simulink model "f22pil"  (Simulink 3.00)
settings: Solver=ode45  StartTime=data.time(1)  StopTime=data.time(end)  RelTol=1e-3
libraries: smxl x7, pil x2
settings Model: BooleanDataType=on  RTWOptions="-aEnforceIntegerDowncast=1 -aFoldNonRolledExpr=1 -aInlineInvariantSignals=0 -aInlineParameters=0 -aLocalBlockOutputs=1 -aRollThreshold=5 -aZeroInternalMemoryAtStartup=1 -aZeroExternalMemoryAtStartup=1 -aInitFltsAndDblsToZero=1 -aGenerateReport=0 -aGenCodeOnly=0 -aRTWVerbose=1 -aIncludeHyperlinkInReport=0 -aLaunchReport=0 -aForceParamTrailComments=0 -aGenerateComments=1 -aIgnoreCustomStorageClasses=1 -aIncHierarchyInIds=0 -aMaxRTWIdLen=31 -aShowEliminatedStatements=0 -aPrefixModelToSubsysFcnNames=1 -aIncDataTypeInIds=0 -aInsertBlockDesc=0 -aSimulinkBlockComments=1 -aInlinedPrmAccess=\"Literals\"  -aSuppressErrorStatus=0 -aModelReferenceCompliant=1 -aSupportNonInlinedSFcns=1 -aSupportContinuousTime=1 -aSupportComplex=1 -aSupportNonFinite=1 -aSupportAbsoluteTime=1 -aTargetFcnLib=\"ansi_tfl_tmw.mat\" -aMultiInstanceERTCode=0 -aLogVarNameModifier=\"rt_\" -aIsPILTarget=0 -aCombineOutputUpdateFcns=0 -aGenerateASAP2=0 -aGenerateSampleERTMain=0 -aGenerateFullHeader=1 -aUtilityFuncGeneration=\"Auto\" -aIncludeFileDelimiter=\"Auto\" -aIncludeMdlTerminateFcn=1 -aPurelyIntegerCode=0 -aERTCustomFileBanners=0 -aRTWCAPIStates=0 -aRTWCAPIParams=0 -aRTWCAPISignals=0 -aMatFileLogging=1 -aGenFloatMathFcnCalls=\"ANSI_C\" -aExtModeMexFile=\"ext_comm\" -aExtModeTransport=0 -aExtModeStaticAllocSize=1000000 -aExtModeTesting=0 -aExtModeStaticAlloc=0 -aExtMode=0"  ExtModeTrigMode=normal  ExtModeArmWhenConnect=on  Creator=Karebear  LastModifiedBy=sim

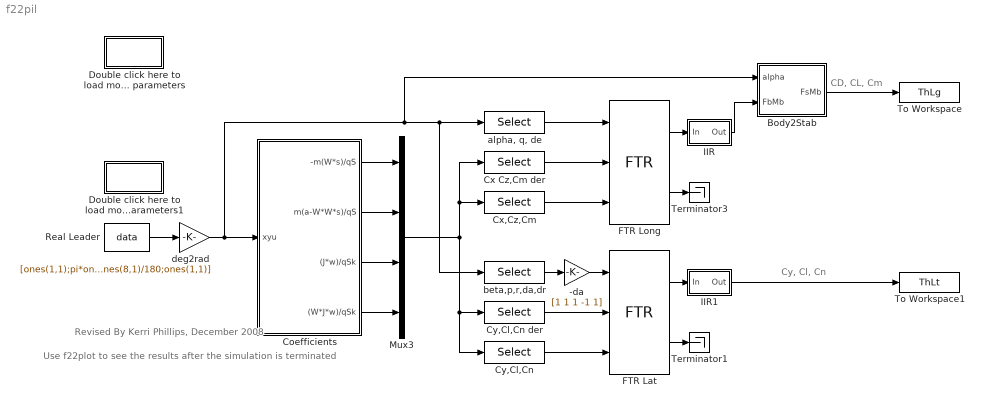
== system f22pil ==
  note: CD, CL, Cm
  note: Cy, Cl, Cn
  note: Revised By Kerri Phillips,
      | December 2008
  note: Use f22plot to see the results
      | after the simulation is terminated
  -da : Gain  Gain=[1 1 1 -1 1]  SaturateOnIntegerOverflow=on
  Body2Stab : Subsystem
  Coefficients : Subsystem
  Cx Cz,Cm der : Selector  Elements=[1 3 8]  InputPortWidth=12
  Cx,Cz,Cm : Selector  Elements=[4 6 11]  InputPortWidth=12
  Cy,Cl,Cn : Selector  Elements=[5 10 12]  InputPortWidth=12
  Cy,Cl,Cn der : Selector  Elements=[2 7 9]  InputPortWidth=12
  Double click here to load model and parameters : Subsystem
      settings: OpenFcn=load f22data;
      mask Display: disp('Load\nData')
  Double click here to load model and parameters1 : Subsystem
      mask Display: disp('Signals')
  FTR Lat : pil/Theta & Cov/FTR  ths=[5 3]  w=2*pi*linspace(0.2,2,30)'  T=0.02
  FTR Long : pil/Theta & Cov/FTR  ths=[3 3]  w=2*pi*linspace(0.2,2,30)'  T=0.02
  IIR : Subsystem  mask(Discrete Time First Order IIR){ni=3*3, a=1, x0=0, T=0.02}
      mask prompts: ni "Number of Channels"; a "Cutoff Frequency (a)"; x0 "Initial Condition"; T "Sample Time"
      mask help:
      | Each channel has the transfer function
      |   (1-exp(-aT))/(1-exp(-aT)(z^-1)) which is a
      |   good approximation of a/(s+a) if 4*pi*a*T<1
      mask init:
      | A=[];B=[];C=[];D=[];
      | for i=1:ni,
      | A=[A,zeros(size(A,1),1);zeros(1,size(A,2)),exp(-a*T)];
      | B=[B,zeros(size(B,1),1);zeros(1,size(B,2)),1-exp(-a*T)];
      | C=[C,zeros(size(C,1),1);zeros(1,size(C,2)),exp(-a*T)];
      | D=[D,zeros(size(D,1),1);zeros(1,size(D,2)),1-exp(-a*T)];
      | end
      mask Help:
      | <p>
      |   Each channel has the transfer function
      |   (1-exp(-aT))/(1-exp(-aT)(z^-1)) which is a
      |   good approximation of a/(s+a) if 4*pi*a*T<1
      | </p>
      mask Display: disp('a/(s+a)')
  IIR1 : Subsystem  mask(Discrete Time First Order IIR){ni=5*3, a=1, x0=0, T=0.02}
      mask prompts: ni "Number of Channels"; a "Cutoff Frequency (a)"; x0 "Initial Condition"; T "Sample Time"
      mask help:
      | Each channel has the transfer function
      |   (1-exp(-aT))/(1-exp(-aT)(z^-1)) which is a
      |   good approximation of a/(s+a) if 4*pi*a*T<1
      mask init: same as f22pil/IIR
      mask Help:
      | <p>
      |   Each channel has the transfer function
      |   (1-exp(-aT))/(1-exp(-aT)(z^-1)) which is a
      |   good approximation of a/(s+a) if 4*pi*a*T<1
      | </p>
      mask Display: disp('a/(s+a)')
  Mux3 : Mux  Inputs=[3 3 3 3]
  Real Leader : FromWorkspace  VariableName=data  SampleTime=0.02  HoldFinalValue=off
  Terminator1 : Terminator
  Terminator3 : Terminator
  To Workspace : ToWorkspace  VariableName=ThLg  SampleTime=0.02  SaveFormat=Matrix
      settings: Buffer=1000
  To Workspace1 : ToWorkspace  VariableName=ThLt  SampleTime=0.02  SaveFormat=Matrix
      settings: Buffer=1000
  "alpha, q, de" : Selector  Elements=[2 5 19]  InputPortWidth=27
  beta,p,r,da,dr : Selector  Elements=[3 4 6 21 23]  InputPortWidth=27
  deg2rad : Gain  Gain=[ones(1,1);pi*ones(8,1)/180;ones(9,1);pi*ones(8,1)/180;ones(1,1)]  SaturateOnIntegerOverflow=on
  wires:
  Real Leader/1 -> deg2rad/1
  deg2rad/1 -> Coefficients/1(xyu), "alpha, q, de"/1, beta,p,r,da,dr/1, Body2Stab/1(alpha)
  "alpha, q, de"/1 -> FTR Long/1
  Cx Cz,Cm der/1 -> FTR Long/2
  Cx,Cz,Cm/1 -> FTR Long/3
  Coefficients/1(-m(W*s)/qS) -> Mux3/1
  Coefficients/2(m(a-W*W*s)/qS) -> Mux3/2
  Coefficients/3((J*w)/qSk) -> Mux3/3
  Coefficients/4((W*J*w)/qSk) -> Mux3/4
  Cy,Cl,Cn der/1 -> FTR Lat/2
  Cy,Cl,Cn/1 -> FTR Lat/3
  Mux3/1 -> Cx Cz,Cm der/1, Cx,Cz,Cm/1, Cy,Cl,Cn/1, Cy,Cl,Cn der/1
  beta,p,r,da,dr/1 -> -da/1
  FTR Long/2 -> Terminator3/1
  FTR Lat/2 -> Terminator1/1
  FTR Long/1 -> IIR/1(In)
  FTR Lat/1 -> IIR1/1(In)
  IIR1/1(Out) -> To Workspace1/1
  -da/1 -> FTR Lat/1
  Body2Stab/1(FsMb) -> To Workspace/1
  IIR/1(Out) -> Body2Stab/2(FbMb)

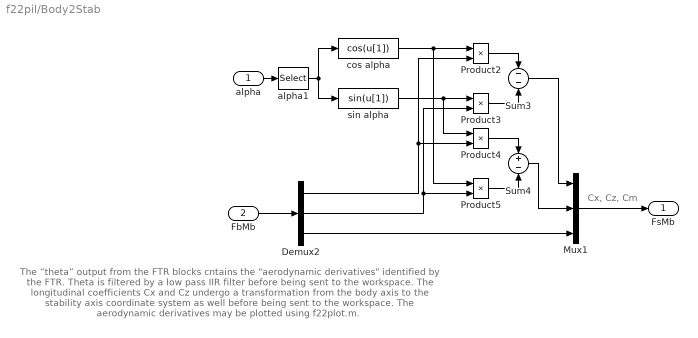
== system f22pil/Body2Stab ==
  note: Cx, Cz, Cm
  note: The “theta” output from the FTR blocks cntains the "aerodynamic derivatives" identified by the FTR.
      | Theta is filtered by a low pass IIR filter before being sent to the workspace.
      | The longitudinal coefficients Cx and Cz undergo a transformation from the body axis
      | to the stability axis coordinate system as well before being sent to the workspace.
      | The aerodynamic derivatives may be plotted using f22plot.m.
  alpha : Inport  Port=1  PortWidth=-1  SampleTime=-1  DataType=auto
      settings: SignalType=auto
  FbMb : Inport  Port=2  PortWidth=-1  SampleTime=-1  DataType=auto
      settings: SignalType=auto
  Demux2 : Demux  Outputs=[3 3 3]
  Mux1 : Mux  Inputs=[3 3 3]
      settings: DisplayOption=none
  Product{2..5} (4 alike) : Product  Inputs=2  SaturateOnIntegerOverflow=on
  Sum3 : Sum  Inputs=--  SaturateOnIntegerOverflow=on
  Sum4 : Sum  Inputs=+-  SaturateOnIntegerOverflow=on
  alpha1 : Selector  Elements=2  InputPortWidth=27
  cos alpha : Fcn  Expr=cos(u[1])
  sin alpha : Fcn  Expr=sin(u[1])
  FsMb : Outport  Port=1
  wires:
  Mux1/1 -> FsMb/1
  Product5/1 -> Sum4/2
  Product4/1 -> Sum4/1
  Demux2/2 -> Product5/2, Product3/2
  sin alpha/1 -> Product4/1, Product3/1
  Product3/1 -> Sum3/2
  Product2/1 -> Sum3/1
  Demux2/1 -> Product4/2, Product2/2
  cos alpha/1 -> Product5/1, Product2/1
  alpha/1 -> alpha1/1
  Sum4/1 -> Mux1/2
  Sum3/1 -> Mux1/1
  Demux2/3 -> Mux1/3
  FbMb/1 -> Demux2/1
  alpha1/1 -> cos alpha/1, sin alpha/1

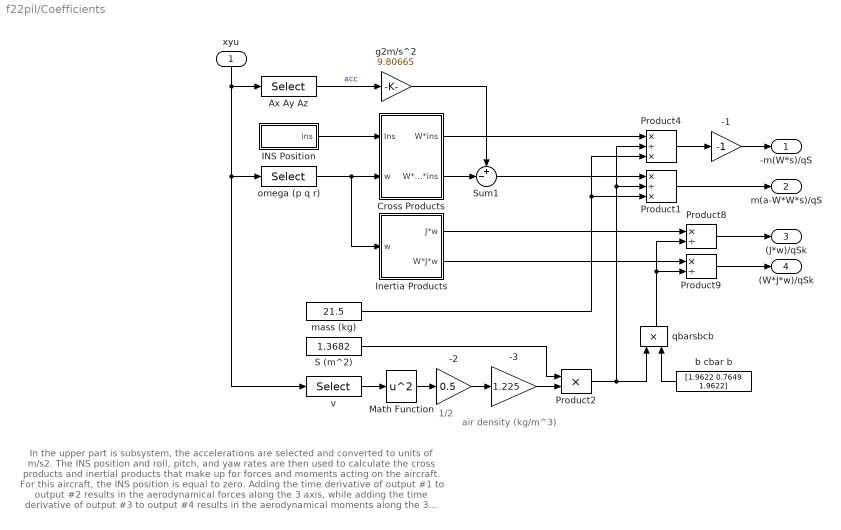
== system f22pil/Coefficients ==
  note: air density
      |  (kg/m^3)
  note: 1/2
  note: In the upper part is subsystem, the accelerations are selected and converted to units of m/s2.
      | The INS position and roll, pitch, and yaw rates are then used to calculate the cross products and inertial products that
      | make up for forces and moments acting on the aircraft. For this aircraft, the INS position is equal to zero.
      | Adding the time derivative of output #1 to output #2 results in the aerodynamical forces along the 3 axis,
      | while adding the time derivative of output #3 to output #4 results in the aerodynamical moments along the 3 axis.
  xyu : Inport  Orientation=down  Port=1  PortWidth=-1  SampleTime=-1  DataType=auto
      settings: SignalType=auto
  -1 : Gain  Gain=-1  SaturateOnIntegerOverflow=on
  -2 : Gain  Gain=0.5  SaturateOnIntegerOverflow=on
  -3 : Gain  Gain=1.225  SaturateOnIntegerOverflow=on
  Ax Ay Az : Selector  Elements=[16 17 18]  InputPortWidth=27
  Cross Products : Subsystem
  INS Position : Subsystem  mask(INS Position in Body Axes){inspos=[0 0 0], cgpos=[0 0 0]}
      mask prompts: inspos "INS Position in inches [FS,BL,WL]"; cgpos "CG  Position in inches [FS,BL,WL]"
      mask help:
      | This block gives in output the INS
      |   position in feets in body axes.
      |
      |   Both INS and CG positions are given
      |   in the mask as Fuselage Station, Butt Line,
      |   and Water Line measurements in inches.
      mask Help:
      | This block gives in output the INS
      |   position in feets in body axes.
      | 
      |   Both INS and CG positions are given
      |   in the mask as Fuselage Station, Butt Line,
      |   and Water Line measurements in inches.
  Inertia Products : Subsystem
  Math Function : Math  Operator=square  OutputSignalType=auto
  Product1 : Product  Inputs=*/*  SaturateOnIntegerOverflow=on
  Product2 : Product  Inputs=**  SaturateOnIntegerOverflow=on
  Product4 : Product  Inputs=*/*  SaturateOnIntegerOverflow=on
  Product8 : Product  Inputs=*/  SaturateOnIntegerOverflow=on
  Product9 : Product  Inputs=*/  SaturateOnIntegerOverflow=on
  S (m^2) : Constant  Value=1.3682
  Sum1 : Sum  Inputs=+-|  SaturateOnIntegerOverflow=on
  b cbar b : Constant  Orientation=left  Value="[1.9622    0.7649    1.9622]"
  g2m/s^2 : Gain  Gain=9.80665  SaturateOnIntegerOverflow=on
  mass (kg) : Constant  Value=21.5
  omega (p q r) : Selector  Elements=[4 5 6]  InputPortWidth=27
  qbarsbcb : Product  Orientation=up  Inputs=2  SaturateOnIntegerOverflow=on
  v : Selector  Elements=1  InputPortWidth=27
  -m(W*s)/qS : Outport  Port=1
  m(a-W*W*s)/qS : Outport  Port=2
  (J*w)/qSk : Outport  Port=3
  (W*J*w)/qSk : Outport  Port=4
  wires:
  Inertia Products/1(J*w) -> Product8/1
  Inertia Products/2(W*J*w) -> Product9/1
  Cross Products/2(W*W*ins) -> Sum1/2
  Product9/1 -> (W*J*w)/qSk/1
  Product8/1 -> (J*w)/qSk/1
  Product4/1 -> -1/1
  -1/1 -> -m(W*s)/qS/1
  Product1/1 -> m(a-W*W*s)/qS/1
  Sum1/1 -> Product1/1
  omega (p q r)/1 -> Inertia Products/1(w), Cross Products/2(w)
  Ax Ay Az/1 -> g2m/s^2/1  "acc"
  INS Position/1(ins) -> Cross Products/1(Ins)
  xyu/1 -> Ax Ay Az/1, omega (p q r)/1, v/1
  Cross Products/1(W*ins) -> Product4/1
  g2m/s^2/1 -> Sum1/1
  mass (kg)/1 -> Product4/3, Product1/3
  S (m^2)/1 -> Product2/1
  v/1 -> Math Function/1
  -2/1 -> -3/1
  Math Function/1 -> -2/1
  -3/1 -> Product2/2
  Product2/1 -> Product4/2, Product1/2, qbarsbcb/1
  qbarsbcb/1 -> Product8/2, Product9/2
  b cbar b/1 -> qbarsbcb/2

== system f22pil/Double click here to load model and parameters ==

== system f22pil/Double click here to load model and parameters1 ==
  note: 1.  Airspeed (m/s)
      | 2.  Angle of Attack (deg)
      | 3.  Sideslip Angle (deg)
      | 4.  Roll Rate (deg/s)
      | 5.  Pitch Rate (deg/s)
      | 6.  Yaw Rate (deg/s)
      | 7.  Yaw Angle (deg)
      | 8.  Pitch Angle (deg)
      | 9.  Roll Angle (deg)
      | 10 x GPS position (m)
      | 11. y GPS position (m)
      | 12. z GPS position (m)
      | 13. x GPS velocity (m/s)
      | 14. y GPS velocity (m/s)
      | 15. z GPS velocity (m/s)
      | 16. x Acceleration (g)
      | 17. y Acceleration (g)
      | 18. z Acceleration (g)
      | 19. Left Stabilator Deflection (deg)
      | 20. Right Stabilator Deflection (deg)
      | 21. Left Aileron Deflection (deg)
      | 22. Right Aileron Deflection (deg)
      | 23. Left Rudder Deflection (deg)
      | 24. Right Rudder Deflection (deg)
      | 25. Left Flap Deflection (deg)
      | 26. Right Flap Deflection (deg)
      | 27.Throttle Command

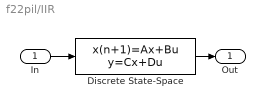
== system f22pil/IIR ==
  In : Inport  Port=1  PortWidth=-1  SampleTime=-1  DataType=auto
      settings: SignalType=auto
  Discrete State-Space : DiscreteStateSpace  A=A  B=B  C=C  D=D  X0=x0  SampleTime=T
  Out : Outport  Port=1
  wires:
  Discrete State-Space/1 -> Out/1
  In/1 -> Discrete State-Space/1

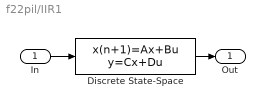
== system f22pil/IIR1 ==
  In : Inport  Port=1  PortWidth=-1  SampleTime=-1  DataType=auto
      settings: SignalType=auto
  Discrete State-Space : DiscreteStateSpace  A=A  B=B  C=C  D=D  X0=x0  SampleTime=T
  Out : Outport  Port=1
  wires:
  In/1 -> Discrete State-Space/1
  Discrete State-Space/1 -> Out/1

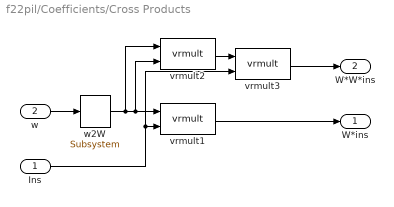
== system f22pil/Coefficients/Cross Products ==
  Ins : Inport  Port=1  PortWidth=-1  SampleTime=-1  DataType=auto
      settings: SignalType=auto
  w : Inport  Port=2  PortWidth=-1  SampleTime=-1  DataType=auto
      settings: SignalType=auto
  vrmult1 : smxl/Real Matrices/vrmult  dims=[3 3 1]
  vrmult2 : smxl/Real Matrices/vrmult  dims=[3 3 3]
  vrmult3 : smxl/Real Matrices/vrmult  dims=[3 3 1]
  w2W : smxl/Rotation Matrices/Quaternions/Body2Earth/Subsystem
  W*ins : Outport  Port=1
  W*W*ins : Outport  Port=2
  wires:
  Ins/1 -> vrmult3/2, vrmult1/2
  vrmult3/1 -> W*W*ins/1
  vrmult2/1 -> vrmult3/1
  vrmult1/1 -> W*ins/1
  w2W/1 -> vrmult2/2, vrmult1/1, vrmult2/1
  w/1 -> w2W/1

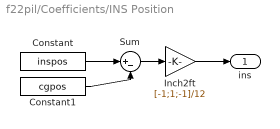
== system f22pil/Coefficients/INS Position ==
  Constant : Constant  Value=inspos
  Constant1 : Constant  Value=cgpos
  Inch2ft : Gain  Gain=[-1;1;-1]/12  SaturateOnIntegerOverflow=on
  Sum : Sum  Inputs=|+-  SaturateOnIntegerOverflow=on
  ins : Outport  Port=1
  wires:
  Inch2ft/1 -> ins/1
  Sum/1 -> Inch2ft/1
  Constant1/1 -> Sum/2
  Constant/1 -> Sum/1

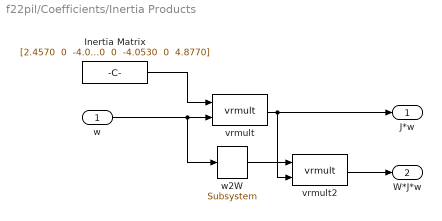
== system f22pil/Coefficients/Inertia Products ==
  w : Inport  Port=1  PortWidth=-1  SampleTime=-1  DataType=auto
      settings: SignalType=auto
  Inertia Matrix : Constant  Value="[2.4570  0  -4.0530  0  6.4810  0  -4.0530  0  4.8770]"
  vrmult : smxl/Real Matrices/vrmult  dims=[3 3 1]
  vrmult2 : smxl/Real Matrices/vrmult  dims=[3 3 1]
  w2W : smxl/Rotation Matrices/Quaternions/Body2Earth/Subsystem
  J*w : Outport  Port=1
  W*J*w : Outport  Port=2
  wires:
  Inertia Matrix/1 -> vrmult/1
  vrmult2/1 -> W*J*w/1
  vrmult/1 -> vrmult2/2, J*w/1
  w2W/1 -> vrmult2/1
  w/1 -> w2W/1, vrmult/2
